simulink model "main_multicore"  (R2017a)
settings: Solver=VariableStepAuto  StartTime=0.0  StopTime=10.0  RelTol=1e-3
libraries: sharedutil x6
settings Model: Creator=hp  LastModifiedBy=hp

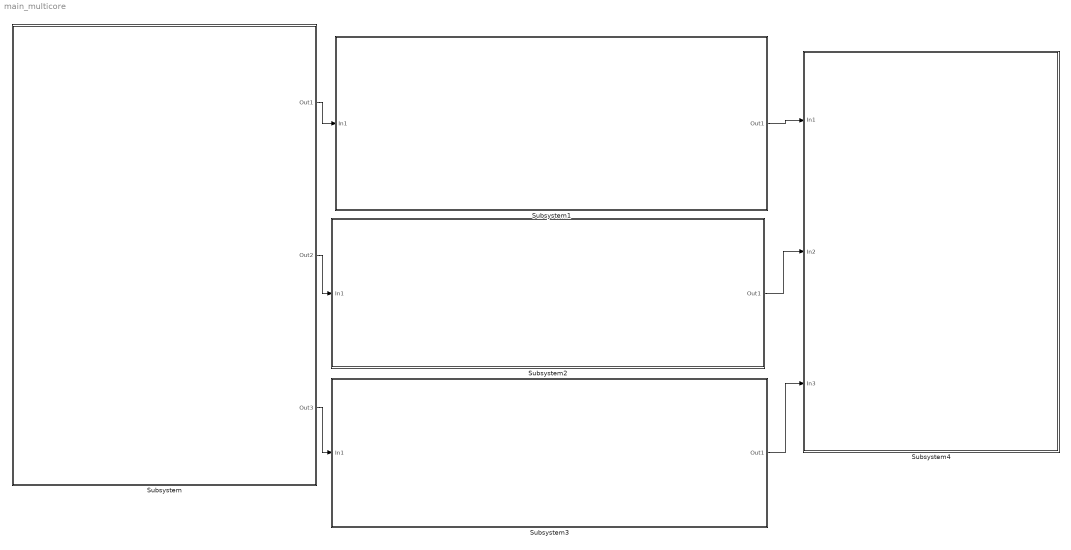
== system main_multicore ==
  Subsystem : Subsystem
  Subsystem1 : Subsystem
  Subsystem2 : Subsystem
  Subsystem3 : Subsystem
  Subsystem4 : Subsystem
  wires:
  Subsystem/1(Out1) -> Subsystem1/1(In1)
  Subsystem/2(Out2) -> Subsystem2/1(In1)
  Subsystem/3(Out3) -> Subsystem3/1(In1)
  Subsystem1/1(Out1) -> Subsystem4/1(In1)
  Subsystem2/1(Out1) -> Subsystem4/2(In2)
  Subsystem3/1(Out1) -> Subsystem4/3(In3)

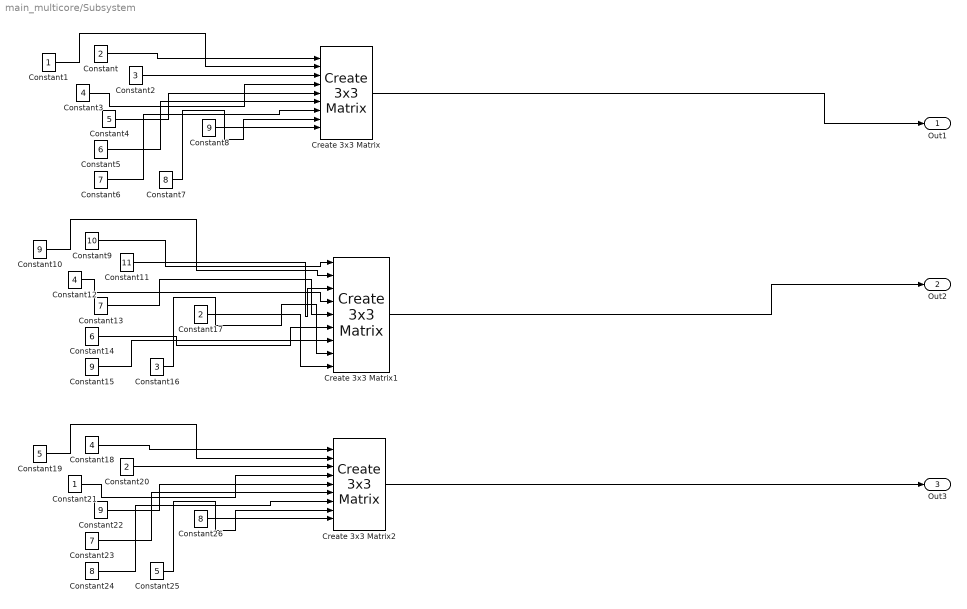
== system main_multicore/Subsystem ==
  Constant : Constant  Value=2
  Constant1 : Constant
  Constant{8,10,15,22} (4 alike) : Constant  Value=9
  Constant11 : Constant  Value=11
  Constant12 : Constant  Value=4
  Constant13 : Constant  Value=7
  Constant14 : Constant  Value=6
  Constant16 : Constant  Value=3
  Constant17 : Constant  Value=2
  Constant18 : Constant  Value=4
  Constant19 : Constant  Value=5
  Constant2 : Constant  Value=3
  Constant20 : Constant  Value=2
  Constant21 : Constant
  Constant23 : Constant  Value=7
  Constant24 : Constant  Value=8
  Constant25 : Constant  Value=5
  Constant26 : Constant  Value=8
  Constant3 : Constant  Value=4
  Constant4 : Constant  Value=5
  Constant5 : Constant  Value=6
  Constant6 : Constant  Value=7
  Constant7 : Constant  Value=8
  Constant9 : Constant  Value=10
  Create 3x3 Matrix : sharedutil/Create 3x3 Matrix
  Create 3x3 Matrix1 : sharedutil/Create 3x3 Matrix
  Create 3x3 Matrix2 : sharedutil/Create 3x3 Matrix
  Out1 : Outport
  Out2 : Outport  Port=2
  Out3 : Outport  Port=3
  wires:
  Constant22/1 -> Create 3x3 Matrix2/5
  Constant15/1 -> Create 3x3 Matrix1/7
  Constant11/1 -> Create 3x3 Matrix1/3
  Constant13/1 -> Create 3x3 Matrix1/5
  Constant16/1 -> Create 3x3 Matrix1/8
  Constant25/1 -> Create 3x3 Matrix2/8
  Constant17/1 -> Create 3x3 Matrix1/9
  Constant23/1 -> Create 3x3 Matrix2/6
  Constant18/1 -> Create 3x3 Matrix2/1
  Constant12/1 -> Create 3x3 Matrix1/4
  Constant9/1 -> Create 3x3 Matrix1/1
  Constant14/1 -> Create 3x3 Matrix1/6
  Constant20/1 -> Create 3x3 Matrix2/3
  Constant10/1 -> Create 3x3 Matrix1/2
  Constant19/1 -> Create 3x3 Matrix2/2
  Constant24/1 -> Create 3x3 Matrix2/7
  Constant21/1 -> Create 3x3 Matrix2/4
  Constant26/1 -> Create 3x3 Matrix2/9
  Constant4/1 -> Create 3x3 Matrix/5
  Constant8/1 -> Create 3x3 Matrix/9
  Constant7/1 -> Create 3x3 Matrix/8
  Constant3/1 -> Create 3x3 Matrix/4
  Constant/1 -> Create 3x3 Matrix/1
  Constant1/1 -> Create 3x3 Matrix/2
  Constant5/1 -> Create 3x3 Matrix/6
  Constant2/1 -> Create 3x3 Matrix/3
  Constant6/1 -> Create 3x3 Matrix/7
  Create 3x3 Matrix/1 -> Out1/1
  Create 3x3 Matrix2/1 -> Out3/1
  Create 3x3 Matrix1/1 -> Out2/1

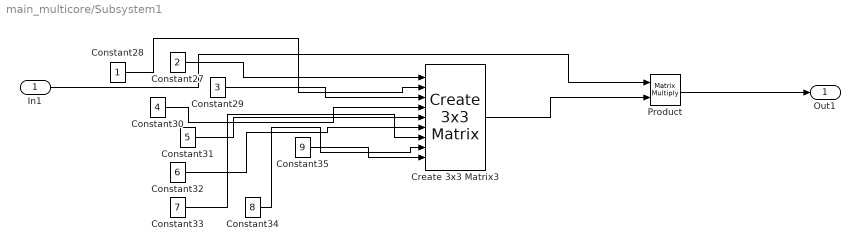
== system main_multicore/Subsystem1 ==
  In1 : Inport
  Constant27 : Constant  Value=2
  Constant28 : Constant
  Constant29 : Constant  Value=3
  Constant30 : Constant  Value=4
  Constant31 : Constant  Value=5
  Constant32 : Constant  Value=6
  Constant33 : Constant  Value=7
  Constant34 : Constant  Value=8
  Constant35 : Constant  Value=9
  Create 3x3 Matrix3 : sharedutil/Create 3x3 Matrix
  Product : Product  Multiplication=Matrix(*)
  Out1 : Outport
  wires:
  Constant32/1 -> Create 3x3 Matrix3/6
  Constant34/1 -> Create 3x3 Matrix3/8
  Constant27/1 -> Create 3x3 Matrix3/1
  Constant31/1 -> Create 3x3 Matrix3/5
  Constant35/1 -> Create 3x3 Matrix3/9
  Constant28/1 -> Create 3x3 Matrix3/2
  Constant33/1 -> Create 3x3 Matrix3/7
  Constant30/1 -> Create 3x3 Matrix3/4
  Constant29/1 -> Create 3x3 Matrix3/3
  Create 3x3 Matrix3/1 -> Product/2
  In1/1 -> Product/1
  Product/1 -> Out1/1

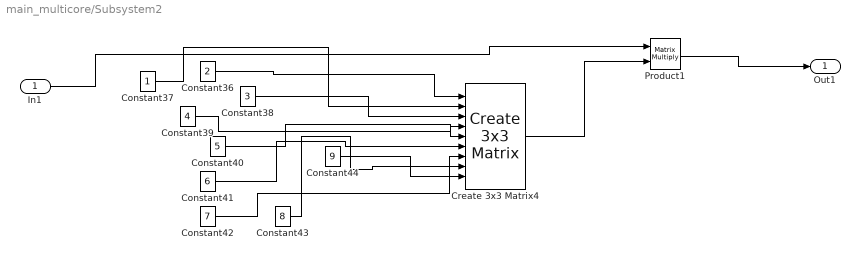
== system main_multicore/Subsystem2 ==
  In1 : Inport
  Constant36 : Constant  Value=2
  Constant37 : Constant
  Constant38 : Constant  Value=3
  Constant39 : Constant  Value=4
  Constant40 : Constant  Value=5
  Constant41 : Constant  Value=6
  Constant42 : Constant  Value=7
  Constant43 : Constant  Value=8
  Constant44 : Constant  Value=9
  Create 3x3 Matrix4 : sharedutil/Create 3x3 Matrix
  Product1 : Product  Multiplication=Matrix(*)
  Out1 : Outport
  wires:
  Product1/1 -> Out1/1
  In1/1 -> Product1/1
  Create 3x3 Matrix4/1 -> Product1/2
  Constant38/1 -> Create 3x3 Matrix4/3
  Constant37/1 -> Create 3x3 Matrix4/2
  Constant43/1 -> Create 3x3 Matrix4/8
  Constant41/1 -> Create 3x3 Matrix4/6
  Constant36/1 -> Create 3x3 Matrix4/1
  Constant42/1 -> Create 3x3 Matrix4/7
  Constant40/1 -> Create 3x3 Matrix4/5
  Constant39/1 -> Create 3x3 Matrix4/4
  Constant44/1 -> Create 3x3 Matrix4/9

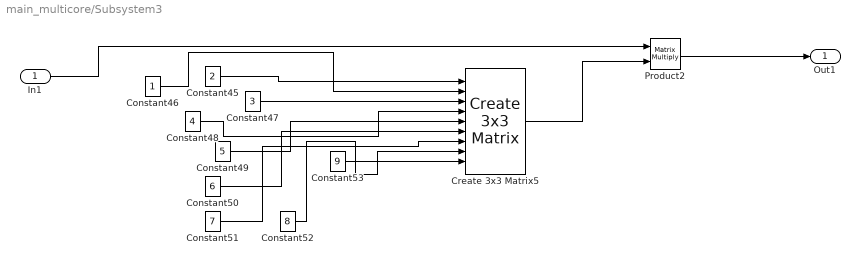
== system main_multicore/Subsystem3 ==
  In1 : Inport
  Constant45 : Constant  Value=2
  Constant46 : Constant
  Constant47 : Constant  Value=3
  Constant48 : Constant  Value=4
  Constant49 : Constant  Value=5
  Constant50 : Constant  Value=6
  Constant51 : Constant  Value=7
  Constant52 : Constant  Value=8
  Constant53 : Constant  Value=9
  Create 3x3 Matrix5 : sharedutil/Create 3x3 Matrix
  Product2 : Product  Multiplication=Matrix(*)
  Out1 : Outport
  wires:
  Create 3x3 Matrix5/1 -> Product2/2
  Product2/1 -> Out1/1
  In1/1 -> Product2/1
  Constant45/1 -> Create 3x3 Matrix5/1
  Constant52/1 -> Create 3x3 Matrix5/8
  Constant47/1 -> Create 3x3 Matrix5/3
  Constant50/1 -> Create 3x3 Matrix5/6
  Constant53/1 -> Create 3x3 Matrix5/9
  Constant46/1 -> Create 3x3 Matrix5/2
  Constant51/1 -> Create 3x3 Matrix5/7
  Constant49/1 -> Create 3x3 Matrix5/5
  Constant48/1 -> Create 3x3 Matrix5/4

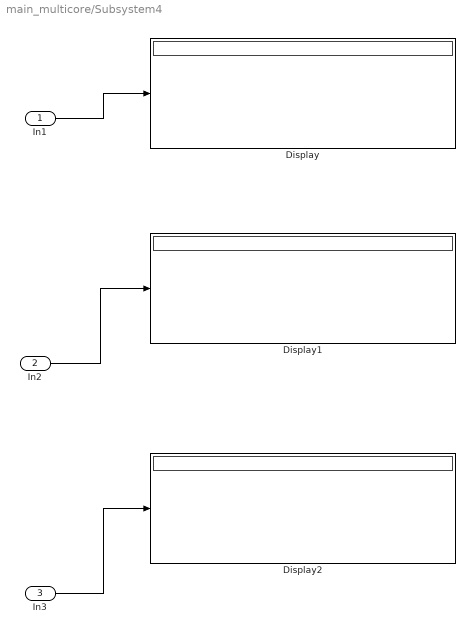
== system main_multicore/Subsystem4 ==
  In1 : Inport
  In2 : Inport  Port=2
  In3 : Inport  Port=3
  Display : Display
  Display1 : Display
  Display2 : Display
  wires:
  In1/1 -> Display/1
  In2/1 -> Display1/1
  In3/1 -> Display2/1
